simulink library "HDL_ieee_8021513"  (R2024a)
settings: Solver=FixedStepDiscrete  StartTime=0.0  StopTime=10.0  RelTol=1e-3
undefined symbols (not defined in the file or in its folder): Add, axiWidth, channelCyclicPrefixLen, channelDataCarriers, channelEstReference, channelLUT, channelOFDMSamples, channelScramblerInit, decimatorDelay, decimatorFilter, fPHY, frequencyOffsetTimeWindow, fs, headerBitsPerFec, headerBitsPerOFDMSymbol, headerBitsPerSubcarrier, headerCyclicPrefixLen, headerDataCarriers, headerOFDMSamples, headerScramblerInit, interpolatorDelay, interpolatorFilter, leftGuard, N, ncoCarrierFrequency, ncoWordLength, numDataCarriers, oversamplingFactor, payloadBitsPerFec, payloadScramblerInit, payloadWordsPerBlock0, peakDetectorThreshold, peakDetectorWindow, preambleCyclicPrefixLen, preambleDataCarriers, preambleLUT, preambleOFDMSamples, preambleScramblerInit, QAM, rightGuard, Shift
libraries: hdlsllib x198, $bdroot x80, whdlutilities x28, whdledac x10, whdlmod x7, simulink x4, dsphdlfiltering2 x2, dsphdlsigops2 x2, commhdlcrc x2, dspsigops x2, dspstat3 x2, commdigbbndam3 x2
(part 4 of 5)

== system HDL_ieee_8021513/full_rx/header_clock_x2 ==
  data_in : Inport
  valid_header : Inport  Port=2
  Demux : Demux
  Serializer1D : hdlsllib/HDL Operations/Serializer1D  Ratio=2  IdleCycles=0  validIn=on  startOut=off  validOut=on  inputDataDimensions=-1  inputSampleTime=-1  inputSignalType=auto
  Terminator : Terminator
  Terminator1 : Terminator
  Vector Concatenate : Concatenate  Mode=Multidimensional array  ConcatenateDimension=2
  rising_edge_detector : $bdroot/rising_edge_detector  SystemSampleTime=-1  VariantActivationTime=update diagram  AllowFlexibleInterface=on  Latency=0  AutoFrameSizeCalculation=off
  data_out : Outport
  start : Outport  Port=2
  wires:
  rising_edge_detector/1 -> start/1
  valid_header/1 -> Serializer1D/2
  data_in/1 -> Demux/1
  Demux/1 -> Terminator/1
  Demux/2 -> Terminator1/1
  Demux/3 -> Vector Concatenate/1
  Demux/4 -> Vector Concatenate/2
  Serializer1D/1 -> data_out/1
  Serializer1D/2 -> rising_edge_detector/1
  Vector Concatenate/1 -> Serializer1D/1

== system HDL_ieee_8021513/full_rx/prepare_payload_data ==
  note: Note_ this counter makes sure that the fifo always has data, and is not emptied in the middle of an LDPC block
  note: Maximum value is 3741
  data_in : Inport
  valid_payload : Inport  Port=2
  payload_ready : Inport  Port=3
  Delay : Delay  DelayLength=1  InitialCondition=0  UseCircularBuffer=on
  Delay2 : Delay  DelayLength=1  InitialCondition=0  UseCircularBuffer=on
  HDL Counter1 : hdlsllib/Sources/HDL Counter  CountType=Count limited  CountInit=0  CountStep=1  CountMax=10000  CountFromType=Initial value  CountFrom=0  CountResetPort=off  CountLoadPort=off  CountEnbPort=on  CountDirPort=off  CountHitOutputPort=on  CountDataType=Unsigned  CountWordLen=14  CountFracLen=0  CountSampTime=1
  HDL FIFO : hdlsllib/HDL RAMs/HDL FIFO  fifo_size=4096  mode=Classic  ratio=1/2  push_msg=Error  pop_msg=Error  show_empty=on  show_full=off  show_num=on  LabelModeActiveChoice_Mode=Classic  rst_port=off
  Logical Operator2 : Logic  IconShape=distinctive  AllPortsSameDT=off  OutDataTypeStr=boolean
  Logical Operator3 : Logic  Operator=NOT  IconShape=distinctive  AllPortsSameDT=off  OutDataTypeStr=boolean
  OR1 : Logic  Operator=OR  IconShape=distinctive  AllPortsSameDT=off  OutDataTypeStr=boolean
  Switch1 : Switch  Criteria=u2 ~= 0  SaturateOnIntegerOverflow=off  InputSameDT=off
  Terminator : Terminator
  Terminator1 : Terminator
  Unit Delay1 : UnitDelay  SampleTime=-1  HasFrameUpgradeWarning=on
  falling_edge_detector1 : $bdroot/falling_edge_detector  SystemSampleTime=-1  VariantActivationTime=update diagram  AllowFlexibleInterface=on  Latency=0  AutoFrameSizeCalculation=off
  payload_clock_x2 : Subsystem
  rising_edge_detector1 : $bdroot/rising_edge_detector  SystemSampleTime=-1  VariantActivationTime=update diagram  AllowFlexibleInterface=on  Latency=0  AutoFrameSizeCalculation=off
  dataOut : Outport
  valid_in : Outport  Port=2
  last_frame : Outport  Port=3
  new_frame : Outport  Port=4
  wires:
  HDL FIFO/3 -> Terminator/1  "fifo_count"
  Delay2/1 -> OR1/2
  HDL Counter1/1 -> Terminator1/1
  OR1/1 -> Switch1/2
  falling_edge_detector1/1 -> OR1/1, Switch1/1
  rising_edge_detector1/1 -> last_frame/1
  HDL Counter1/2 -> Delay2/1, new_frame/1  "new_frame"
  Unit Delay1/1 -> Switch1/3
  Switch1/1 -> HDL Counter1/1, Unit Delay1/1
  HDL FIFO/2 -> Logical Operator3/1, falling_edge_detector1/1, rising_edge_detector1/1  "fifo_empty"
  data_in/1 -> payload_clock_x2/1(data_in)
  payload_clock_x2/2(valid_out) -> HDL FIFO/2  "push"
  payload_clock_x2/1(data_out) -> HDL FIFO/1  "dataIn"
  HDL FIFO/1 -> dataOut/1  "dataOut"
  valid_payload/1 -> payload_clock_x2/2(valid_in)
  Logical Operator2/1 -> HDL FIFO/3, Delay/1
  Delay/1 -> valid_in/1  "valid_in"
  Logical Operator3/1 -> Logical Operator2/1
  payload_ready/1 -> Logical Operator2/2  "payload_ready"

== system HDL_ieee_8021513/full_tx/FIFO ==
  preamble : Inport
  preamble_valid : Inport  Port=2
  channel : Inport  Port=3
  channel_valid : Inport  Port=4
  header : Inport  Port=5
  header_valid : Inport  Port=6
  payload : Inport  Port=7
  payload_valid : Inport  Port=8
  payload_len : Inport  Port=9
  bits_per_subcarrier : Inport  Port=10
  cp_len_in : Inport  Port=11
  ready : Inport  Port=12
  Delay : Delay  DelayLength=1  InitialCondition=0  UseCircularBuffer=on
  HDL FIFO : hdlsllib/HDL RAMs/HDL FIFO  fifo_size=65536  mode=Classic  ratio=1  push_msg=Warning  pop_msg=Warning  show_empty=on  show_full=on  show_num=on  LabelModeActiveChoice_Mode=Classic  rst_port=off
  data_out : Outport
  valid_out : Outport  Port=2
  bits_per_subcarrier_out : Outport  Port=3
  init : Outport  Port=4
  new : Outport  Port=5
  cp_len : Outport  Port=6
  wires:
  Delay/1 -> valid_out/1
  HDL FIFO/1 -> data_out/1
  ready/1 -> HDL FIFO/3, Delay/1

== system HDL_ieee_8021513/full_tx/clock_crossing ==
  preamble_in : Inport
  preamble_ctrl_in : Inport  Port=2
  channel : Inport  Port=3
  channel_ctrl : Inport  Port=4
  header_in : Inport  Port=5
  header_ctrl_in : Inport  Port=6
  payload_in : Inport  Port=7
  payload_ctrl_in : Inport  Port=8
  cp_len_in : Inport  Port=9
  payload_len_in : Inport  Port=10
  bits_per_subcarrier_in : Inport  Port=11
  Deserializer1D : hdlsllib/HDL Operations/Deserializer1D  Ratio=2  IdleCycles=0  InitialCondition=0  startIn=off  validIn=on  validOut=on  inputDataDimensions=-1  inputSampleTime=-1  inputSignalType=auto
  Deserializer1D1 : hdlsllib/HDL Operations/Deserializer1D  Ratio=2  IdleCycles=0  InitialCondition=0  startIn=off  validIn=on  validOut=on  inputDataDimensions=-1  inputSampleTime=-1  inputSignalType=auto
  Rate Transition : RateTransition  OutPortSampleTime=1/fPHY
  Rate Transition1 : RateTransition  OutPortSampleTime=1/fPHY
  Rate Transition2 : RateTransition  OutPortSampleTime=1/fPHY
  Sample Control Bus Selector{,1..3} (4 alike) : whdlutilities/Sample Control Bus Selector  OutputSignals=start,end,valid
  Terminator{,1..7} (8 alike) : Terminator
  preamble_out : Outport
  preamble_valid : Outport  Port=2
  channel_out : Outport  Port=3
  channel_valid : Outport  Port=4
  header_out : Outport  Port=5
  header_valid : Outport  Port=6
  payload_out : Outport  Port=7
  payload_valid_out : Outport  Port=8
  payload_len_out : Outport  Port=9  VectorParamsAs1DForOutWhenUnconnected=off
  bits_per_subcarrier_out : Outport  Port=10  VectorParamsAs1DForOutWhenUnconnected=off
  cp_len_out : Outport  Port=11  VectorParamsAs1DForOutWhenUnconnected=off
  wires:
  preamble_ctrl_in/1 -> Sample Control Bus Selector/1
  Sample Control Bus Selector/1 -> Terminator/1
  Sample Control Bus Selector/2 -> Terminator1/1
  Sample Control Bus Selector/3 -> preamble_valid/1
  preamble_in/1 -> preamble_out/1
  Sample Control Bus Selector1/3 -> channel_valid/1
  channel_ctrl/1 -> Sample Control Bus Selector1/1
  Sample Control Bus Selector1/2 -> Terminator3/1
  Sample Control Bus Selector1/1 -> Terminator2/1
  channel/1 -> channel_out/1
  Sample Control Bus Selector2/1 -> Terminator5/1
  Deserializer1D/1 -> header_out/1
  Sample Control Bus Selector2/2 -> Terminator4/1
  Deserializer1D/2 -> header_valid/1
  header_ctrl_in/1 -> Sample Control Bus Selector2/1
  Sample Control Bus Selector2/3 -> Deserializer1D/2
  header_in/1 -> Deserializer1D/1
  Sample Control Bus Selector3/1 -> Terminator7/1
  Deserializer1D1/2 -> payload_valid_out/1
  Sample Control Bus Selector3/2 -> Terminator6/1
  payload_ctrl_in/1 -> Sample Control Bus Selector3/1
  Deserializer1D1/1 -> payload_out/1
  Sample Control Bus Selector3/3 -> Deserializer1D1/2
  payload_in/1 -> Deserializer1D1/1
  bits_per_subcarrier_in/1 -> Rate Transition2/1
  payload_len_in/1 -> Rate Transition1/1
  cp_len_in/1 -> Rate Transition/1
  Rate Transition/1 -> cp_len_out/1
  Rate Transition1/1 -> payload_len_out/1
  Rate Transition2/1 -> bits_per_subcarrier_out/1

== system HDL_ieee_8021513/full_tx/new_frame_rate_conversion ==
  note: Description:
      | This block "extends" the "end" signal 4 clock cycles, to ensure that the "end" signal can be sampled by the rate transition block.
      | (Otherwise, the "end" signal would be "on" only 1/4th of a cycle, and it can't be ensured that it will be read).
  ctrl_in : Inport
  Delay2 : Delay  DelayLength=1  InitialCondition=0  UseCircularBuffer=on
  Delay3 : Delay  DelayLength=1  InitialCondition=0  UseCircularBuffer=on
  Delay4 : Delay  DelayLength=1  InitialCondition=0  UseCircularBuffer=on
  Logical Operator : Logic  Operator=OR  Inputs=4  IconShape=distinctive  AllPortsSameDT=off  OutDataTypeStr=boolean
  Rate Transition2 : RateTransition  OutPortSampleTime=1/(fPHY/4)
  Sample Control Bus Selector1 : whdlutilities/Sample Control Bus Selector  OutputSignals=start,end,valid
  Terminator2 : Terminator
  Terminator3 : Terminator
  new_frame : Outport  VectorParamsAs1DForOutWhenUnconnected=off
  wires:
  Logical Operator/1 -> Rate Transition2/1
  Sample Control Bus Selector1/3 -> Terminator2/1
  Delay2/1 -> Logical Operator/2, Delay3/1
  Delay3/1 -> Logical Operator/3, Delay4/1
  Sample Control Bus Selector1/2 -> Logical Operator/1, Delay2/1
  Delay4/1 -> Logical Operator/4
  Sample Control Bus Selector1/1 -> Terminator3/1
  ctrl_in/1 -> Sample Control Bus Selector1/1
  Rate Transition2/1 -> new_frame/1

== system HDL_ieee_8021513/full_tx/new_frame_rate_conversion1 ==
  note: Description:
      | This block "extends" the "end" signal 8 clock cycles, to ensure that the "end" signal can be sampled by the rate transition block.
      | (Otherwise, the "end" signal would be "on" only 1/4th of a cycle, and it can't be ensured that it will be read).
  ctrl_in : Inport
  Delay{1..7} (7 alike) : Delay  DelayLength=1  InitialCondition=0  UseCircularBuffer=on
  Logical Operator : Logic  Operator=OR  Inputs=8  IconShape=distinctive  AllPortsSameDT=off  OutDataTypeStr=boolean
  Rate Transition2 : RateTransition  OutPortSampleTime=1/(fPHY/4)
  Sample Control Bus Selector1 : whdlutilities/Sample Control Bus Selector  OutputSignals=start,end,valid
  Terminator2 : Terminator
  Terminator3 : Terminator
  new_frame : Outport  VectorParamsAs1DForOutWhenUnconnected=off
  wires:
  Logical Operator/1 -> Rate Transition2/1
  Sample Control Bus Selector1/3 -> Terminator2/1
  Delay2/1 -> Logical Operator/2, Delay3/1
  Delay3/1 -> Logical Operator/3, Delay4/1
  Sample Control Bus Selector1/2 -> Logical Operator/1, Delay2/1
  Delay4/1 -> Logical Operator/8, Delay1/1
  Sample Control Bus Selector1/1 -> Terminator3/1
  ctrl_in/1 -> Sample Control Bus Selector1/1
  Rate Transition2/1 -> new_frame/1
  Delay1/1 -> Logical Operator/7, Delay5/1
  Delay5/1 -> Logical Operator/6, Delay6/1
  Delay6/1 -> Logical Operator/5, Delay7/1
  Delay7/1 -> Logical Operator/4

== system HDL_ieee_8021513/full_tx/store_frame_in_ram ==
  preamble : Inport
  preamble_valid : Inport  Port=2
  channel : Inport  Port=3
  channel_valid : Inport  Port=4
  header : Inport  Port=5
  header_valid : Inport  Port=6
  payload : Inport  Port=7
  payload_valid : Inport  Port=8
  payload_len : Inport  Port=9
  bits_per_subcarrier : Inport  Port=10
  cp_len_in : Inport  Port=11
  ready : Inport  Port=12
  Delay : Delay  DelayLength=1  InitialCondition=0  UseCircularBuffer=on
  RAM : Subsystem
  Switch1 : Switch  Criteria=u2 ~= 0  SaturateOnIntegerOverflow=off  InputSameDT=off
  Unit Delay1 : UnitDelay  SampleTime=-1  HasFrameUpgradeWarning=on
  read_frame_from_ram : Subsystem
  write_frame_to_ram : Subsystem
  data_out : Outport
  valid_out : Outport  Port=2
  bits_per_subcarrier_out : Outport  Port=3
  init : Outport  Port=4
  new : Outport  Port=5
  cp_len : Outport  Port=6
  wires:
  read_frame_from_ram/1(rd_addr) -> RAM/4(new_rd_addr)  "new_rd_addr"
  bits_per_subcarrier/1 -> read_frame_from_ram/3(bits_per_subcarrier)
  header/1 -> write_frame_to_ram/5(header)
  write_frame_to_ram/1(write_data) -> RAM/1(new_din)  "new_din"
  write_frame_to_ram/4(end) -> read_frame_from_ram/1(start_reading)
  cp_len_in/1 -> read_frame_from_ram/4(cp_len_in)
  Switch1/1 -> Unit Delay1/1, data_out/1  "dout_magic"
  write_frame_to_ram/3(we) -> RAM/3(new_we)  "new_we"
  ready/1 -> read_frame_from_ram/Enable, Delay/1
  Delay/1 -> Switch1/2
  preamble/1 -> write_frame_to_ram/1(preamble)
  channel_valid/1 -> write_frame_to_ram/4(channel_valid)
  read_frame_from_ram/3(bits_per_subcarrier_out) -> bits_per_subcarrier_out/1
  payload/1 -> write_frame_to_ram/7(payload)
  RAM/1(dout_new) -> Switch1/1
  read_frame_from_ram/5(new) -> new/1  "new_new"
  read_frame_from_ram/4(init) -> init/1
  write_frame_to_ram/5(ram_size) -> read_frame_from_ram/2(ram_size)
  preamble_valid/1 -> write_frame_to_ram/2(preamble_valid)
  Unit Delay1/1 -> Switch1/3
  payload_len/1 -> write_frame_to_ram/9(payload_len)
  channel/1 -> write_frame_to_ram/3(channel)
  write_frame_to_ram/2(wr_addr) -> RAM/2(new_wr_addr)  "new_wr_addr"
  read_frame_from_ram/2(valid_out) -> valid_out/1  "valid_new"
  payload_valid/1 -> write_frame_to_ram/8(payload_valid)
  header_valid/1 -> write_frame_to_ram/6(header_valid)
  read_frame_from_ram/6(cp_len) -> cp_len/1

== system HDL_ieee_8021513/ldpc_encoder/output_selector ==
  codeRate : Inport
  blockSize : Inport  Port=2
  Buffer1 : $bdroot/Buffer  SystemSampleTime=-1  VariantActivationTime=update diagram  AllowFlexibleInterface=on  Latency=0  AutoFrameSizeCalculation=off
  Demux2 : Demux  Outputs=2
  Demux3 : Demux  Outputs=3
  Logical Operator3 : Logic  IconShape=distinctive  AllPortsSameDT=off  OutDataTypeStr=boolean
  Logical Operator5 : Logic  Operator=OR  IconShape=distinctive  AllPortsSameDT=off  OutDataTypeStr=boolean
  Logical Operator6 : Logic  IconShape=distinctive  AllPortsSameDT=off  OutDataTypeStr=boolean
  Logical Operator7 : Logic  Operator=NOT  IconShape=distinctive  AllPortsSameDT=off  OutDataTypeStr=boolean
  Terminator1 : Terminator
  m2 : Outport  VectorParamsAs1DForOutWhenUnconnected=off
  m1 : Outport  Port=2  VectorParamsAs1DForOutWhenUnconnected=off
  m0 : Outport  Port=3  VectorParamsAs1DForOutWhenUnconnected=off
  wires:
  Buffer1/1 -> m0/1  "Out0"
  Logical Operator6/1 -> m1/1  "Out1"
  codeRate/1 -> Demux3/1
  blockSize/1 -> Demux2/1
  Demux2/1 -> Buffer1/1  "K0"
  Demux3/1 -> Logical Operator3/2, Logical Operator7/1  "R0"
  Logical Operator5/1 -> m2/1  "Out2"
  Logical Operator7/1 -> Logical Operator6/1
  Demux3/2 -> Logical Operator6/2, Logical Operator3/1  "R1"
  Demux2/2 -> Terminator1/1  "K1"
  Logical Operator3/1 -> Logical Operator5/1
  Demux3/3 -> Logical Operator5/2  "R2"

== system HDL_ieee_8021513/ofdm_separator/wait_for_header ==
  note: Store payload OFDM symbols until header parameters are known (cyclic prefix has to be known before demodulating the OFDM symbol)
  note: The RAM value should be large enough to wait for the header to be processed.
      | Th e LDPC decoder of the header has a delay > 2500, so a value of 3000 is chosen for an extra margin.
  data_in : Inport
  header_ready : Inport  Port=2
  valid_payload : Inport  Port=3
  zero_payload : Inport  Port=4
  one_payload : Inport  Port=5
  ofdm_samples : Inport  Port=6
  AND : Logic  IconShape=distinctive  AllPortsSameDT=off  OutDataTypeStr=boolean
  Delay12 : Delay  DelayLength=1  InitialCondition=0  UseCircularBuffer=on
  Delay13 : Delay  DelayLength=1  InitialCondition=0  UseCircularBuffer=on
  Delay14 : Delay  DelayLength=1  InitialCondition=0  UseCircularBuffer=on
  HDL Counter : hdlsllib/Sources/HDL Counter  CountType=Free running  CountInit=0  CountStep=1  CountMax=25  CountFromType=Initial value  CountFrom=0  CountResetPort=on  CountLoadPort=off  CountEnbPort=on  CountDirPort=off  CountHitOutputPort=off  CountDataType=Unsigned  CountWordLen=16  CountFracLen=0  CountSampTime=1
  HDL FIFO : hdlsllib/HDL RAMs/HDL FIFO  fifo_size=2100  mode=Classic  ratio=1  push_msg=Error  pop_msg=Error  show_empty=on  show_full=off  show_num=on  LabelModeActiveChoice_Mode=Classic  rst_port=on
  Logical Operator1 : Logic  Operator=OR  Inputs=3  IconShape=distinctive  AllPortsSameDT=off  OutDataTypeStr=boolean
  NOT : Logic  Operator=NOT  IconShape=distinctive  AllPortsSameDT=off  OutDataTypeStr=boolean
  OR : Logic  Operator=OR  IconShape=distinctive  AllPortsSameDT=off  OutDataTypeStr=boolean
  OR2 : Logic  Operator=OR  IconShape=distinctive  AllPortsSameDT=off  OutDataTypeStr=boolean
  Relational Operator : RelationalOperator  Operator===  OutDataTypeStr=boolean  RndMeth=Simplest  InputSameDT=off
  Switch : Switch  Criteria=u2 ~= 0  SaturateOnIntegerOverflow=off  InputSameDT=off
  Switch3 : Switch  Criteria=u2 ~= 0  SaturateOnIntegerOverflow=off  InputSameDT=off
  Terminator : Terminator
  Unit Delay : UnitDelay  SampleTime=-1  HasFrameUpgradeWarning=on
  rising_edge_detector : $bdroot/rising_edge_detector  SystemSampleTime=-1  VariantActivationTime=update diagram  AllowFlexibleInterface=on  Latency=0  AutoFrameSizeCalculation=off
  rising_edge_detector1 : $bdroot/rising_edge_detector  SystemSampleTime=-1  VariantActivationTime=update diagram  AllowFlexibleInterface=on  Latency=0  AutoFrameSizeCalculation=off
  data_out : Outport
  valid_payload_out : Outport  Port=2
  wires:
  Delay13/1 -> HDL FIFO/2
  data_in/1 -> Switch3/3, Delay12/1
  Delay12/1 -> HDL FIFO/1
  valid_payload/1 -> Delay13/1, rising_edge_detector1/1
  Switch3/1 -> data_out/1
  HDL FIFO/2 -> [empty]
  HDL FIFO/1 -> Switch3/1
  rising_edge_detector1/1 -> OR/1
  zero_payload/1 -> OR/2
  HDL FIFO/3 -> Terminator/1  "fifo_ofdm"
  [empty] -> rising_edge_detector/1
  rising_edge_detector/1 -> Logical Operator1/1
  Unit Delay/1 -> Switch/3
  Switch/1 -> Delay14/1, HDL FIFO/3, Unit Delay/1  "pop"
  Logical Operator1/1 -> Switch/2
  header_ready/1 -> HDL Counter/1, Switch/1, Logical Operator1/2
  HDL Counter/1 -> Relational Operator/1  "count"
  ofdm_samples/1 -> Relational Operator/2
  OR/1 -> OR2/1
  Relational Operator/1 -> OR2/2, NOT/1, Logical Operator1/3  "hit_zero"
  OR2/1 -> HDL FIFO/4
  one_payload/1 -> HDL Counter/2
  AND/1 -> Switch3/2, valid_payload_out/1
  Delay14/1 -> AND/1
  NOT/1 -> AND/2

== system HDL_ieee_8021513/ofdm_symbol_sync/find_peak ==
  data_in : Inport
  M_in : Inport  Port=2
  Compare To Constant : hdlsllib/Logic and Bit Operations/Compare To Constant  relop=>  const=peakDetectorThreshold  OutDataTypeStr=boolean
  Constant : Constant  Value=0  OutDataTypeStr=Inherit: Inherit via back propagation  SampleTime=-1
  Delay{,1..4} (5 alike) : Delay  DelayLength=1  InitialCondition=0  UseCircularBuffer=on
  Delay5 : Delay  DelayLength=peakDetectorWindow-1  InitialCondition=0  UseCircularBuffer=on
  HDL Counter : hdlsllib/Sources/HDL Counter  CountType=Count limited  CountInit=0  CountStep=1  CountMax=peakDetectorWindow-1  CountFromType=Initial value  CountFrom=0  CountResetPort=on  CountLoadPort=off  CountEnbPort=on  CountDirPort=off  CountHitOutputPort=on  CountDataType=Unsigned  CountWordLen=nextpow2(peakDetectorWindow)  CountFracLen=0  CountSampTime=1
  OR : Logic  Operator=OR  IconShape=distinctive  AllPortsSameDT=off  OutDataTypeStr=boolean
  OR1 : Logic  Operator=OR  IconShape=distinctive  AllPortsSameDT=off  OutDataTypeStr=boolean
  Relational Operator : RelationalOperator  Operator=>  OutDataTypeStr=boolean  InputSameDT=off
  Switch : Switch  Criteria=u2 ~= 0  SaturateOnIntegerOverflow=off
  Switch1 : Switch  Criteria=u2 ~= 0  SaturateOnIntegerOverflow=off
  Switch2 : Switch  Criteria=u2 ~= 0  SaturateOnIntegerOverflow=off  InputSameDT=off
  Terminator : Terminator
  Unit Delay : UnitDelay  SampleTime=-1  HasFrameUpgradeWarning=on
  Unit Delay1 : UnitDelay  SampleTime=-1  HasFrameUpgradeWarning=on
  data_out : Outport  VectorParamsAs1DForOutWhenUnconnected=off
  peak_sync : Outport  Port=2  VectorParamsAs1DForOutWhenUnconnected=off
  wires:
  M_in/1 -> Switch1/1, Compare To Constant/1  "data_in"
  Unit Delay/1 -> Switch/3
  Switch/1 -> Unit Delay/1, Relational Operator/2  "peak(i)"
  Relational Operator/1 -> HDL Counter/1, Delay3/1  "new_peak"
  Switch1/1 -> Delay2/1  "peak(i+1)"
  Constant/1 -> Switch1/3
  Unit Delay1/1 -> Switch2/3
  Switch2/1 -> Unit Delay1/1, HDL Counter/2  "en"
  HDL Counter/2 -> Delay1/1, peak_sync/1
  OR/1 -> Switch2/2
  [new_peak] -> OR/2
  [peak_found] -> OR/1
  HDL Counter/1 -> Terminator/1
  Delay/1 -> Switch/1
  Delay1/1 -> [peak_found]  "peak_found"
  OR1/1 -> Switch/2
  [new_peak] -> OR1/1
  [peak_found] -> OR1/2
  Delay3/1 -> [new_peak], Switch2/1
  Compare To Constant/1 -> Switch1/2
  Delay2/1 -> Delay/1, Relational Operator/1
  data_in/1 -> Delay4/1
  Delay4/1 -> Delay5/1
  Delay5/1 -> data_out/1

== system HDL_ieee_8021513/ofdm_symbol_sync/frequency_offset_calculator ==
  peak_sync : Inport
  P(d) : Inport  Port=2
  Complex to Magnitude-Angle : dsphdlmathfun2/Complex to Magnitude-Angle  NumIterationsSource=Auto  NumIterations=10  OutputFormat=Angle  AngleFormat=Radians  ScaleOutput=off  ScalingMethod=Shift-Add  SimulateUsing=Code generation
  Delay : Delay  InitialCondition=0  UseCircularBuffer=on
  Delay1 : Delay  InitialCondition=0  UseCircularBuffer=on
  Gain : Gain  Gain=fi(1/(pi*frequencyOffsetTimeWindow), 0, 32, 16)  ParamDataTypeStr=fixdt(0,32,16)  OutDataTypeStr=fixdt(1,32,16)
  Switch : Switch  Criteria=u2 ~= 0  SaturateOnIntegerOverflow=off  InputSameDT=off
  Unit Delay : UnitDelay  SampleTime=-1  HasFrameUpgradeWarning=on
  frequency_offset : Outport
  wires:
  Switch/1 -> Unit Delay/1, frequency_offset/1
  Unit Delay/1 -> Switch/3
  Delay/1 -> Switch/1
  Delay1/1 -> Switch/2
  Gain/1 -> Delay/1
  Complex to Magnitude-Angle/1 -> Gain/1
  P(d)/1 -> Complex to Magnitude-Angle/1
  peak_sync/1 -> Complex to Magnitude-Angle/2
  Complex to Magnitude-Angle/2 -> Delay1/1

== system HDL_ieee_8021513/ofdm_symbol_sync/m_cox ==
  note: Latency of the real divide block is:
      |
      | 1 + nextpow2(u.WordLength + 1 - issigned(u) + 1) + 2 + u.WordLength + 2 - issigned(u) + 5
  note: Delay of m_cox = delay blocks + delay divider + delay_10_preambles_symbols
      | Delay of m_cox = 5 + 47 + 2580
  data_in : Inport
  Compare To Zero : hdlsllib/Logic and Bit Operations/Compare To Zero  relop=~=  OutDataTypeStr=boolean
  Constant : Constant  OutDataTypeStr=boolean  SampleTime=-1
  Constant1 : Constant  OutDataTypeStr=Inherit: Inherit via back propagation  SampleTime=-1
  Data Type Conversion1 : DataTypeConversion  OutDataTypeStr=fixdt(1,32,24)  SaturateOnIntegerOverflow=off  RndMeth=Floor
  Delay1 : Delay  DelayLength=47  InitialCondition=0  UseCircularBuffer=on
  Delay4 : Delay  DelayLength=(N+preambleCyclicPrefixLen)*10  InitialCondition=0  UseCircularBuffer=on
  Delay5 : Delay  DelayLength=47  InitialCondition=0  UseCircularBuffer=on
  Delay6 : Delay  DelayLength=5  InitialCondition=0  UseCircularBuffer=on
  Real Divide HDL Optimized : embreciprocals/Real Divide HDL Optimized  OutputType=fixdt(1,16,12)
      settings: LibrarySourceBlock=embeddedMatrixLib/Math Operations/Real Divide HDL Optimized
  Switch : Switch  Criteria=u2 ~= 0  SaturateOnIntegerOverflow=off  InputSameDT=off
  Terminator : Terminator
  calculate_P : Subsystem
  calculate_R : Subsystem
  data_out : Outport  VectorParamsAs1DForOutWhenUnconnected=off
  M(d) : Outport  Port=2  VectorParamsAs1DForOutWhenUnconnected=off
  P(d) : Outport  Port=3  VectorParamsAs1DForOutWhenUnconnected=off
  wires:
  Constant/1 -> Real Divide HDL Optimized/3
  data_in/1 -> Delay4/1, Data Type Conversion1/1
  calculate_P/1(|P(d)|2) -> Real Divide HDL Optimized/1  "P"
  Real Divide HDL Optimized/1 -> M(d)/1
  Delay1/1 -> P(d)/1
  Delay6/1 -> Delay5/1
  Delay5/1 -> data_out/1
  Delay4/1 -> Delay6/1
  calculate_P/2(P(d)) -> Delay1/1
  Data Type Conversion1/1 -> calculate_R/1(r(d)), calculate_P/1(r(d))
  Real Divide HDL Optimized/2 -> Terminator/1
  Constant1/1 -> Switch/3
  Compare To Zero/1 -> Switch/2
  Switch/1 -> Real Divide HDL Optimized/2
  calculate_R/1(Rf2) -> Switch/1, Compare To Zero/1  "R"

== system HDL_ieee_8021513/payload_full/psdu_size_to_payload_len ==
  note: Get length of the payload expressed in OFDM Symbols:
      |
      | bitsInPsdu = psduSize * 8 * fecRate [bits/payload]
      | bitsInOFDMSymbol = numDataCarriers * bitsPerSubcarrier [bits/OFDM]
      |
      | payloadLenInOFDMSymbols = ceil( bitsInPsdu / bitsInOFDMSymbol ) [OFDM/payload]
  note: Repetition not supported
  note: Adding "1" is the same as doing a "ceil()" operation,
      | because the divider "floors" the previous result.
      | It is assumed that the division will never be an integer
  bits_per_subcarrier : Inport
  psdu_size : Inport  Port=2
  rep_number : Inport  Port=3
  Add1 : Sum  OutDataTypeStr=Inherit: Same as first input
  Bit Shift : hdlsllib/Logic and Bit Operations/Bit Shift  mode=Shift Left Logical  N=4
  Bit Shift2 : hdlsllib/Logic and Bit Operations/Bit Shift  mode=Shift Right Arithmetic  N=0
  Bit Shift3 : hdlsllib/Logic and Bit Operations/Bit Shift  mode=Shift Right Arithmetic  N=1
  Bit Shift5 : hdlsllib/Logic and Bit Operations/Bit Shift  mode=Shift Right Arithmetic  N=4
  Bits to Word1 : hdlsllib/Logic and Bit Operations/Bits to Word
  Constant4 : Constant  OutDataTypeStr=fixdt(0,1,0)  SampleTime=-1
  Data Type Conversion1 : DataTypeConversion  OutDataTypeStr=fixdt(0,1,0)  SaturateOnIntegerOverflow=off  RndMeth=Floor
  Delay{,1..2,6} (4 alike) : Delay  DelayLength=1  InitialCondition=0  UseCircularBuffer=on
  Gain : Gain  Gain=fi(1/numDataCarriers, 0, 16, 16)  ParamDataTypeStr=fixdt(1,16,15)  OutDataTypeStr=uint16
  Multiport Switch : MultiPortSwitch  DataPortOrder=Zero-based contiguous  Inputs=5  zeroidx=on  SaturateOnIntegerOverflow=off  InputSameDT=off
  Terminator : Terminator
  payload_len_in_ofdm_symbols : Outport
  wires:
  rep_number/1 -> Terminator/1
  bits_per_subcarrier/1 -> Delay1/1
  Data Type Conversion1/1 -> Bits to Word1/1
  Multiport Switch/1 -> Gain/1
  Constant4/1 -> Add1/2
  psdu_size/1 -> Data Type Conversion1/1
  Bits to Word1/1 -> Bit Shift/1
  Add1/1 -> Delay6/1  "payloadNumOFDMSymbols"
  Delay6/1 -> payload_len_in_ofdm_symbols/1
  Bit Shift/1 -> Delay/1
  Bit Shift2/1 -> Multiport Switch/2, Multiport Switch/3
  Bit Shift3/1 -> Multiport Switch/5, Multiport Switch/4
  Bit Shift5/1 -> Multiport Switch/6
  Delay/1 -> Bit Shift2/1, Bit Shift5/1, Bit Shift3/1
  Delay1/1 -> Multiport Switch/1
  Gain/1 -> Delay2/1
  Delay2/1 -> Add1/1

== system HDL_ieee_8021513/peak_detector/local_peak ==
  index : Inport
  dataIn : Inport  Port=2
  AND : Logic  IconShape=distinctive  AllPortsSameDT=off  OutDataTypeStr=boolean
  AND1 : Logic  IconShape=distinctive  AllPortsSameDT=off  OutDataTypeStr=boolean
  AND2 : Logic  IconShape=distinctive  AllPortsSameDT=off  OutDataTypeStr=boolean
  Delay{,1..5} (6 alike) : Delay  DelayLength=1  InitialCondition=0  UseCircularBuffer=on
  HDL Counter : hdlsllib/Sources/HDL Counter  CountType=Count limited  CountInit=0  CountStep=1  CountMax=peakDetectorWindow-1  CountFromType=Initial value  CountFrom=0  CountResetPort=on  CountLoadPort=off  CountEnbPort=on  CountDirPort=off  CountHitOutputPort=on  CountDataType=Unsigned  CountWordLen=nextpow2(peakDetectorWindow+1)  CountFracLen=0  CountSampTime=-1
  NOT : Logic  Operator=NOT  IconShape=distinctive  AllPortsSameDT=off  OutDataTypeStr=boolean
  OR : Logic  Operator=OR  IconShape=distinctive  AllPortsSameDT=off  OutDataTypeStr=boolean
  OR1 : Logic  Operator=OR  IconShape=distinctive  AllPortsSameDT=off  OutDataTypeStr=boolean
  OR2 : Logic  Operator=OR  IconShape=distinctive  AllPortsSameDT=off  OutDataTypeStr=boolean
  Relational Operator : RelationalOperator  OutDataTypeStr=boolean  RndMeth=Simplest  InputSameDT=off
  Switch : Switch  Criteria=u2 ~= 0  SaturateOnIntegerOverflow=off  InputSameDT=off
  Switch1 : Switch  Criteria=u2 ~= 0  SaturateOnIntegerOverflow=off  InputSameDT=off
  Terminator : Terminator
  Unit Delay : UnitDelay  SampleTime=-1  HasFrameUpgradeWarning=on
  Unit Delay1 : UnitDelay  SampleTime=-1  HasFrameUpgradeWarning=on
  peak_sync : Outport
  wires:
  HDL Counter/1 -> Terminator/1  "count"
  Unit Delay/1 -> Switch/3
  Switch/1 -> Relational Operator/2, Unit Delay/1  "dataIn(indexes(i)"
  Unit Delay1/1 -> Switch1/3
  Switch1/1 -> HDL Counter/2, Delay3/1, Unit Delay1/1  "count_enable"
  OR/1 -> Delay4/1
  dataIn/1 -> Relational Operator/1, Delay1/1
  index/1 -> AND1/1  "input"
  Delay4/1 -> Switch1/2  "open"
  Delay5/1 -> Switch1/1  "new_index"
  Delay/1 -> Switch/2
  Delay1/1 -> Switch/1
  Relational Operator/1 -> [higher]
  NOT/1 -> AND1/2
  AND1/1 -> [new_peak], OR1/1
  OR1/1 -> Delay2/1  "rst"
  AND2/1 -> OR1/2
  AND/1 -> OR2/1
  OR2/1 -> Delay/1
  [en] -> NOT/1
  [en] -> AND2/1
  [en] -> AND/1
  Delay3/1 -> [en]
  [higher] -> AND/2
  [higher] -> AND2/2
  [peak_found] -> OR/2
  HDL Counter/2 -> peak_sync/1, [peak_found]  "counter_hit"
  [new_peak] -> Delay5/1
  [new_peak] -> OR/1
  [new_peak] -> OR2/2
  Delay2/1 -> HDL Counter/1  "new_index"

== system HDL_ieee_8021513/peak_detector/s1_index ==
  dataIn : Inport
  Add : Sum
  Bit Shift : hdlsllib/Logic and Bit Operations/Bit Shift  mode=Shift Right Arithmetic  N=1
  Compare To Constant : hdlsllib/Logic and Bit Operations/Compare To Constant  relop=>  const=peakDetectorThreshold  OutDataTypeStr=boolean
  Delay : Delay  DelayLength=peakDetectorWindow  InitialCondition=0  UseCircularBuffer=on
  Delay{1..5} (5 alike) : Delay  DelayLength=1  InitialCondition=0  UseCircularBuffer=on
  Minimum : dspstat3/Minimum  operation=minimum  fcn=Value  indexBase=Zero  operateOver=Each column  Dimension=1  InputProcessing=Columns as channels (frame based)  reset=None  roiEnable=off  roiType=Rectangles  roiPortion=Entire ROI  roiOutput=Individual statistics for each ROI  roiFlag=off  roundingMode=Floor  overflowMode=off
      settings: LibrarySourceBlock=dsphdlsupportstat/Minimum
  Minimum1 : dspstat3/Minimum  operation=minimum  fcn=Value  indexBase=Zero  operateOver=Each column  Dimension=1  InputProcessing=Columns as channels (frame based)  reset=None  roiEnable=off  roiType=Rectangles  roiPortion=Entire ROI  roiOutput=Individual statistics for each ROI  roiFlag=off  roundingMode=Floor  overflowMode=off
      settings: LibrarySourceBlock=dsphdlsupportstat/Minimum
  Tapped Delay : simulink/Discrete/Tapped Delay  vinit=0.0  samptime=-1  NumDelays=peakDetectorWindow  DelayOrder=Oldest  includeCurrent=off
  Tapped Delay1 : simulink/Discrete/Tapped Delay  vinit=0.0  samptime=-1  NumDelays=peakDetectorWindow  DelayOrder=Oldest  includeCurrent=off
  indexes : Outport
  Output : Outport  Port=2
  wires:
  dataIn/1 -> Tapped Delay/1, Delay/1  "x(i+peakDetectorWindow+1)"
  Delay/1 -> Delay2/1  "x(i+1)"
  Tapped Delay/1 -> Minimum/1  "x(i+1:i+peakDetectorWindow)"
  Tapped Delay1/1 -> Minimum1/1  "x(i-peakDetectorWindow:i-1)"
  Minimum/1 -> Add/1  "xmin_new"
  Minimum1/1 -> Add/2  "xmin_bot"
  Bit Shift/1 -> Delay3/1  "s1"
  Delay2/1 -> Delay4/1, Tapped Delay1/1  "x(i)"
  Compare To Constant/1 -> indexes/1
  Add/1 -> Delay1/1
  Delay1/1 -> Bit Shift/1
  Delay3/1 -> Compare To Constant/1
  Delay4/1 -> Delay5/1
  Delay5/1 -> Output/1

== system HDL_ieee_8021513/qam_demod/to_12bit_integer ==
  1bit : Inport
  2bit : Inport  Port=2
  4bit : Inport  Port=3
  Constant{,1..2,12,14} (5 alike) : Constant  Value=0  OutDataTypeStr=Inherit: Inherit via back propagation  SampleTime=-1
  Demux : Demux  Outputs=2
  Demux1 : Demux
  Vector Concatenate : Concatenate  NumInputs=4  Mode=Multidimensional array
  Vector Concatenate1 : Concatenate  NumInputs=4  Mode=Multidimensional array
  Vector Concatenate2 : Concatenate  NumInputs=4  Mode=Multidimensional array
  1bit_out : Outport
  2bit_out : Outport  Port=2
  4bit_out : Outport  Port=3
  wires:
  2bit/1 -> Demux/1
  4bit/1 -> Demux1/1
  Vector Concatenate/1 -> 4bit_out/1
  Vector Concatenate1/1 -> 2bit_out/1
  Vector Concatenate2/1 -> 1bit_out/1
  Constant2/1 -> Vector Concatenate2/1
  Constant1/1 -> Vector Concatenate2/2
  Constant/1 -> Vector Concatenate2/3
  1bit/1 -> Vector Concatenate2/4
  Constant14/1 -> Vector Concatenate1/1
  Constant12/1 -> Vector Concatenate1/2
  Demux/1 -> Vector Concatenate1/3
  Demux/2 -> Vector Concatenate1/4
  Demux1/1 -> Vector Concatenate/1
  Demux1/2 -> Vector Concatenate/2
  Demux1/3 -> Vector Concatenate/3
  Demux1/4 -> Vector Concatenate/4

== system HDL_ieee_8021513/rx_demodulator_full/get_bits_per_subcarrier ==
  payload_bits_per_sub : Inport
  valid_header : Inport  Port=2
  Constant3 : Constant  Value=headerBitsPerSubcarrier  OutDataTypeStr=uint8  SampleTime=-1
  Data Type Conversion2 : DataTypeConversion  OutDataTypeStr=fixdt(0,4,0)  SaturateOnIntegerOverflow=off  RndMeth=Floor
  Data Type Conversion7 : DataTypeConversion  OutDataTypeStr=fixdt(0,4,0)  SaturateOnIntegerOverflow=off  RndMeth=Floor
  Switch1 : Switch  Criteria=u2 ~= 0  SaturateOnIntegerOverflow=off  InputSameDT=off
  qam_demod_bits : Outport
  wires:
  Switch1/1 -> qam_demod_bits/1
  payload_bits_per_sub/1 -> Data Type Conversion2/1
  valid_header/1 -> Switch1/2
  Data Type Conversion2/1 -> Switch1/3
  Constant3/1 -> Data Type Conversion7/1
  Data Type Conversion7/1 -> Switch1/1

== system HDL_ieee_8021513/rx_demodulator_full/get_cp ==
  valid_header : Inport
  valid_payload : Inport  Port=2
  cp_payload : Inport  Port=3
  Bit Concat : hdlsllib/Logic and Bit Operations/Bit Concat  numInputs=2
  Constant : Constant  Value=channelCyclicPrefixLen  OutDataTypeStr=uint8  SampleTime=-1
  Constant1 : Constant  Value=headerCyclicPrefixLen  OutDataTypeStr=uint8  SampleTime=-1
  Data Type Conversion : DataTypeConversion  OutDataTypeStr=uint8  SaturateOnIntegerOverflow=off  RndMeth=Floor
  Data Type Conversion1 : DataTypeConversion  OutDataTypeStr=fixdt(0,2,0)  SaturateOnIntegerOverflow=off  RndMeth=Floor
  Data Type Conversion5 : DataTypeConversion  OutDataTypeStr=uint8  SaturateOnIntegerOverflow=off  RndMeth=Floor
  Data Type Conversion6 : DataTypeConversion  OutDataTypeStr=uint8  SaturateOnIntegerOverflow=off  RndMeth=Floor
  Multiport Switch : MultiPortSwitch  DataPortOrder=Zero-based contiguous  zeroidx=on  SaturateOnIntegerOverflow=off
  ofdm_cp_len : Outport
  wires:
  Data Type Conversion1/1 -> Multiport Switch/1
  valid_header/1 -> Bit Concat/2
  valid_payload/1 -> Bit Concat/1
  Data Type Conversion/1 -> Multiport Switch/4
  Data Type Conversion5/1 -> Multiport Switch/3
  Data Type Conversion6/1 -> Multiport Switch/2
  Multiport Switch/1 -> ofdm_cp_len/1
  cp_payload/1 -> Data Type Conversion/1
  Constant/1 -> Data Type Conversion6/1
  Constant1/1 -> Data Type Conversion5/1
  Bit Concat/1 -> Data Type Conversion1/1  "control"

== system HDL_ieee_8021513/rx_demodulator_full/get_init ==
  valid_header : Inport
  valid_payload : Inport  Port=2
  Bit Concat : hdlsllib/Logic and Bit Operations/Bit Concat  numInputs=2
  Constant4 : Constant  Value=channelScramblerInit  OutDataTypeStr=uint8  SampleTime=-1
  Constant5 : Constant  Value=headerScramblerInit  OutDataTypeStr=uint8  SampleTime=-1
  Constant6 : Constant  Value=payloadScramblerInit  OutDataTypeStr=uint8  SampleTime=-1
  Data Type Conversion10 : DataTypeConversion  OutDataTypeStr=boolean  SaturateOnIntegerOverflow=off  RndMeth=Floor
  Data Type Conversion4 : DataTypeConversion  OutDataTypeStr=boolean  SaturateOnIntegerOverflow=off  RndMeth=Floor
  Data Type Conversion9 : DataTypeConversion  OutDataTypeStr=boolean  SaturateOnIntegerOverflow=off  RndMeth=Floor
  Multiport Switch2 : MultiPortSwitch  DataPortOrder=Zero-based contiguous  zeroidx=on  SaturateOnIntegerOverflow=off  InputSameDT=off
  descrambler_init : Outport
  wires:
  Bit Concat/1 -> Multiport Switch2/1  "control"
  valid_header/1 -> Bit Concat/2
  valid_payload/1 -> Bit Concat/1
  Data Type Conversion10/1 -> Multiport Switch2/2
  Multiport Switch2/1 -> descrambler_init/1
  Constant4/1 -> Data Type Conversion10/1
  Constant5/1 -> Data Type Conversion9/1
  Data Type Conversion4/1 -> Multiport Switch2/4
  Constant6/1 -> Data Type Conversion4/1
  Data Type Conversion9/1 -> Multiport Switch2/3

== system HDL_ieee_8021513/rx_demodulator_full/ofdm_rx_counter ==
  note: Counts the amount of OFDM symbols for every "end" signal, and assigns them a position (preamble, channel, header, payload)
  valid : Inport
  rst : Inport  Port=2
  payload_num_ofdm_symbols : Inport  Port=3
  Add : Sum
  Constant1 : Constant  Value=2  OutDataTypeStr=uint16  SampleTime=-1
  Constant2 : Constant  Value=3  OutDataTypeStr=uint16  SampleTime=-1
  Constant3 : Constant  Value=3  OutDataTypeStr=uint16  SampleTime=-1
  HDL Counter : hdlsllib/Sources/HDL Counter  CountType=Free running  CountInit=0  CountStep=1  CountMax=25  CountFromType=Initial value  CountFrom=0  CountResetPort=on  CountLoadPort=off  CountEnbPort=on  CountDirPort=off  CountHitOutputPort=off  CountDataType=Unsigned  CountWordLen=16  CountFracLen=0  CountSampTime=1
  Logical Operator2 : Logic  IconShape=distinctive  AllPortsSameDT=off  OutDataTypeStr=boolean
  Logical Operator3 : Logic  Operator=NOT  IconShape=distinctive  AllPortsSameDT=off  OutDataTypeStr=boolean
  Logical Operator4 : Logic  Operator=NOT  IconShape=distinctive  AllPortsSameDT=off  OutDataTypeStr=boolean
  Logical Operator5 : Logic  IconShape=distinctive  AllPortsSameDT=off  OutDataTypeStr=boolean
  Relational Operator1 : RelationalOperator  Operator=<  OutDataTypeStr=boolean  InputSameDT=off
  Relational Operator2 : RelationalOperator  Operator=<  OutDataTypeStr=boolean  InputSameDT=off
  Relational Operator3 : RelationalOperator  Operator=<  OutDataTypeStr=boolean  InputSameDT=off
  falling_edge_detector : $bdroot/falling_edge_detector  SystemSampleTime=-1  VariantActivationTime=update diagram  AllowFlexibleInterface=on  Latency=0  AutoFrameSizeCalculation=off
  falling_edge_detector1 : $bdroot/falling_edge_detector  SystemSampleTime=-1  VariantActivationTime=update diagram  AllowFlexibleInterface=on  Latency=0  AutoFrameSizeCalculation=off
  rising_edge_detector1 : $bdroot/rising_edge_detector  SystemSampleTime=-1  VariantActivationTime=update diagram  AllowFlexibleInterface=on  Latency=0  AutoFrameSizeCalculation=off
  is_channel : Outport
  is_header : Outport  Port=2
  is_payload : Outport  Port=3
  last_frame : Outport  Port=4  VectorParamsAs1DForOutWhenUnconnected=off
  wires:
  Relational Operator3/1 -> Logical Operator5/2
  Constant3/1 -> Add/1
  Add/1 -> Relational Operator3/2
  payload_num_ofdm_symbols/1 -> Add/2
  falling_edge_detector/1 -> last_frame/1
  Logical Operator5/1 -> is_payload/1, falling_edge_detector/1  "payload"
  Logical Operator4/1 -> Logical Operator5/1  "payload"
  valid/1 -> falling_edge_detector1/1
  falling_edge_detector1/1 -> HDL Counter/2
  Constant1/1 -> Relational Operator1/2
  Constant2/1 -> Relational Operator2/2
  HDL Counter/1 -> Relational Operator1/1, Relational Operator2/1, Relational Operator3/1
  Relational Operator2/1 -> Logical Operator4/1, Logical Operator2/2
  Logical Operator3/1 -> Logical Operator2/1
  Logical Operator2/1 -> is_header/1  "header"
  Relational Operator1/1 -> Logical Operator3/1, is_channel/1  "channel"
  rst/1 -> rising_edge_detector1/1
  rising_edge_detector1/1 -> HDL Counter/1

== system HDL_ieee_8021513/rx_payload_full/next_frame_to_ready_rx ==
  note: Given a next frame rising edge, this subsystem will generate a "ready" signal for the duration of "payloadBitsPerFec" clock cycles
  next_frame : Inport
  HDL Counter : hdlsllib/Sources/HDL Counter  CountType=Count limited  CountInit=0  CountStep=1  CountMax=payloadBitsPerFec-1  CountFromType=Initial value  CountFrom=0  CountResetPort=off  CountLoadPort=off  CountEnbPort=on  CountDirPort=off  CountHitOutputPort=on  CountDataType=Unsigned  CountWordLen=nextpow2(payloadBitsPerFec)  CountFracLen=0  CountSampTime=1
  Logical Operator2 : Logic  Operator=NOT  IconShape=distinctive  AllPortsSameDT=off  OutDataTypeStr=boolean
  Logical Operator3 : Logic  Operator=OR  IconShape=distinctive  AllPortsSameDT=off  OutDataTypeStr=boolean
  Terminator : Terminator
  Unit Delay Enabled Synchronous : hdlsllib/Discrete/Unit Delay Enabled Synchronous  InitialCondition=0.0  SampleTime=-1
  rising_edge_detector : $bdroot/rising_edge_detector  SystemSampleTime=-1  VariantActivationTime=update diagram  AllowFlexibleInterface=on  Latency=0  AutoFrameSizeCalculation=off
  ready : Outport  VectorParamsAs1DForOutWhenUnconnected=off
  wires:
  rising_edge_detector/1 -> Logical Operator3/1
  Logical Operator2/1 -> Unit Delay Enabled Synchronous/1
  HDL Counter/1 -> Terminator/1
  Unit Delay Enabled Synchronous/1 -> HDL Counter/1, ready/1
  Logical Operator3/1 -> Unit Delay Enabled Synchronous/2
  HDL Counter/2 -> Logical Operator3/2, Logical Operator2/1
  next_frame/1 -> rising_edge_detector/1

== system HDL_ieee_8021513/rx_payload_full/reduced_ldpc_rx ==
  data_in : Inport
  ctrl_in : Inport  Port=2
  fec_rate : Inport  Port=3
  block_size : Inport  Port=4
  Hc_12S_B80 : whdledac/LDPC Decoder  ParityCheckMatrix=Hc_12S  BlockSize=80  Algorithm=Min-sum  ScalingFactor=0.75  Termination=Max  SpecifyInputs=Property  NumIterations=ldpcDecoderMaxNumberIterations  MaxNumIterations=8  ParityCheckStatus=off  SimulateUsing=Code generation
  Terminator : Terminator
  Terminator1 : Terminator
  data_out : Outport
  ctrl_out : Outport  Port=2
  next_frame : Outport  Port=3  VectorParamsAs1DForOutWhenUnconnected=off
  wires:
  Hc_12S_B80/1 -> data_out/1
  Hc_12S_B80/2 -> ctrl_out/1
  data_in/1 -> Hc_12S_B80/1
  ctrl_in/1 -> Hc_12S_B80/2
  fec_rate/1 -> Terminator/1
  block_size/1 -> Terminator1/1
  Hc_12S_B80/3 -> next_frame/1

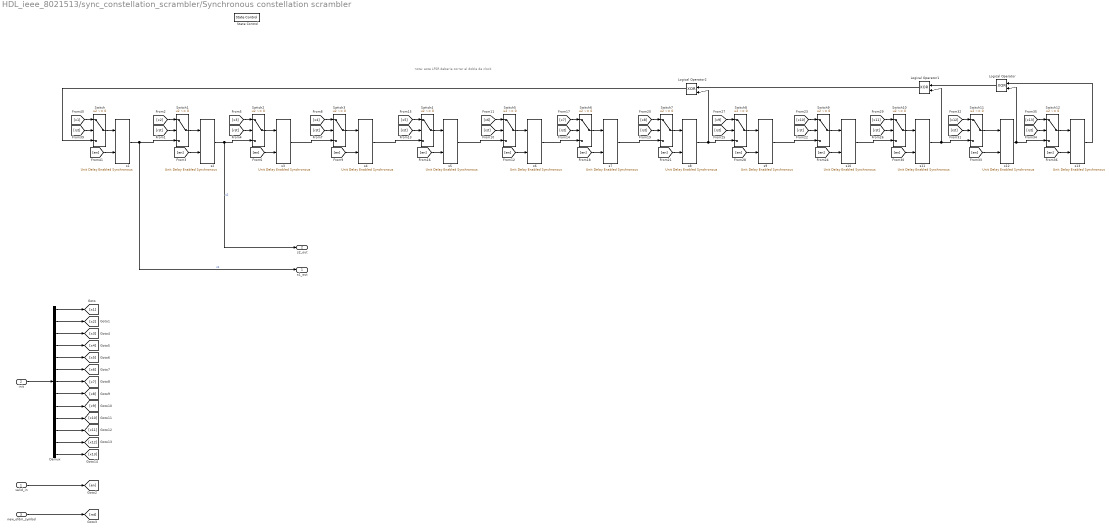
== system HDL_ieee_8021513/sync_constellation_scrambler/Synchronous constellation scrambler ==
  note: nota: este LFSR deberia correr al doble de clock
  valid_in : Inport
  init : Inport  Port=2
  new_ofdm_symbol : Inport  Port=3
  Demux : Demux  Outputs=13
  Logical Operator : Logic  Operator=XOR  IconShape=distinctive  AllPortsSameDT=off  OutDataTypeStr=boolean
  Logical Operator1 : Logic  Operator=XOR  IconShape=distinctive  AllPortsSameDT=off  OutDataTypeStr=boolean
  Logical Operator2 : Logic  Operator=XOR  IconShape=distinctive  AllPortsSameDT=off  OutDataTypeStr=boolean
  State Control : StateControl  StateControl=Synchronous
  Switch{,1..12} (13 alike) : Switch  Criteria=u2 ~= 0  SaturateOnIntegerOverflow=off  InputSameDT=off
  s{1..13} (13 alike) : hdlsllib/Discrete/Unit Delay Enabled Synchronous  InitialCondition=0.0  SampleTime=-1
  s1_out : Outport  VectorParamsAs1DForOutWhenUnconnected=off
  s2_out : Outport  Port=2  VectorParamsAs1DForOutWhenUnconnected=off
  wires:
  [en] -> s11/2
  Demux/5 -> [x5]
  Logical Operator1/1 -> Logical Operator2/1
  [rst] -> Switch2/2
  s3/1 -> Switch3/3
  [rst] -> Switch9/2
  [x5] -> Switch4/1
  s8/1 -> Switch8/3, Logical Operator2/2
  Demux/13 -> [x13]
  [en] -> s9/2
  s13/1 -> Logical Operator/1
  Switch6/1 -> s7/1
  [en] -> s8/2
  [x9] -> Switch8/1
  [x2] -> Switch1/1
  s4/1 -> Switch4/3
  [rst] -> Switch/2
  Switch8/1 -> s9/1
  [x4] -> Switch3/1
  Switch12/1 -> s13/1
  [en] -> s7/2
  init/1 -> Demux/1
  [en] -> s4/2
  Switch7/1 -> s8/1
  s2/1 -> s2_out/1, Switch2/3  "s2"
  [rst] -> Switch11/2
  s9/1 -> Switch9/3
  [en] -> s5/2
  Demux/10 -> [x10]
  [en] -> s12/2
  Switch9/1 -> s10/1
  Switch1/1 -> s2/1
  s12/1 -> Switch12/3, Logical Operator/2
  [x7] -> Switch6/1
  Switch11/1 -> s12/1
  [rst] -> Switch6/2
  [en] -> s3/2
  [en] -> s2/2
  Demux/4 -> [x4]
  [x3] -> Switch2/1
  [en] -> s1/2
  Demux/2 -> [x2]
  valid_in/1 -> [en]
  [en] -> s6/2
  s6/1 -> Switch6/3
  Switch5/1 -> s6/1
  [rst] -> Switch12/2
  [x10] -> Switch9/1
  Logical Operator2/1 -> Switch/3
  [rst] -> Switch7/2
  Demux/11 -> [x11]
  Switch/1 -> s1/1
  Switch4/1 -> s5/1
  [rst] -> Switch5/2
  [x6] -> Switch5/1
  [x11] -> Switch10/1
  Logical Operator/1 -> Logical Operator1/1
  s5/1 -> Switch5/3
  s11/1 -> Switch11/3, Logical Operator1/2
  [x1] -> Switch/1
  Demux/9 -> [x9]
  s10/1 -> Switch10/3
  new_ofdm_symbol/1 -> [rst]
  [rst] -> Switch3/2
  [en] -> s13/2
  [rst] -> Switch1/2
  [x12] -> Switch11/1
  [rst] -> Switch8/2
  [en] -> s10/2
  Switch2/1 -> s3/1
  Demux/3 -> [x3]
  Demux/7 -> [x7]
  [rst] -> Switch4/2
  Demux/8 -> [x8]
  Demux/1 -> [x1]
  Demux/12 -> [x12]
  Demux/6 -> [x6]
  Switch3/1 -> s4/1
  s1/1 -> s1_out/1, Switch1/3  "s1"
  [rst] -> Switch10/2
  [x8] -> Switch7/1
  s7/1 -> Switch7/3
  Switch10/1 -> s11/1
  [x13] -> Switch12/1

== system HDL_ieee_8021513/constellation_descrambler/rotate_-90/rotate_-90 ==
  s2 : Inport
  s1 : Inport  Port=2
  data_in : Inport  Port=3
  Bit Concat : hdlsllib/Logic and Bit Operations/Bit Concat  numInputs=2
  Complex to Real-Imag : ComplexToRealImag
  Complex to Real-Imag1 : ComplexToRealImag
  Complex to Real-Imag2 : ComplexToRealImag
  Multiport Switch : MultiPortSwitch  DataPortOrder=Zero-based contiguous  Inputs=4  zeroidx=on  SaturateOnIntegerOverflow=off  InputSameDT=off
  Real-Imag to Complex : RealImagToComplex
  Real-Imag to Complex1 : RealImagToComplex
  Real-Imag to Complex2 : RealImagToComplex
  Unary Minus{,1..3} (4 alike) : UnaryMinus
  data_out : Outport
  wires:
  Unary Minus3/1 -> Real-Imag to Complex/2
  Multiport Switch/1 -> data_out/1
  Real-Imag to Complex2/1 -> Multiport Switch/5
  Complex to Real-Imag2/1 -> Real-Imag to Complex2/2
  Real-Imag to Complex1/1 -> Multiport Switch/3
  Complex to Real-Imag1/2 -> Real-Imag to Complex1/1
  Real-Imag to Complex/1 -> Multiport Switch/4
  Complex to Real-Imag/2 -> Unary Minus3/1
  Unary Minus/1 -> Real-Imag to Complex/1
  Complex to Real-Imag/1 -> Unary Minus/1
  data_in/1 -> Multiport Switch/2, Complex to Real-Imag/1, Complex to Real-Imag2/1, Complex to Real-Imag1/1
  Bit Concat/1 -> Multiport Switch/1
  s1/1 -> Bit Concat/2
  s2/1 -> Bit Concat/1
  Complex to Real-Imag1/1 -> Unary Minus1/1
  Unary Minus1/1 -> Real-Imag to Complex1/2
  Complex to Real-Imag2/2 -> Unary Minus2/1
  Unary Minus2/1 -> Real-Imag to Complex2/1

== system HDL_ieee_8021513/full_rx/prepare_payload_data/payload_clock_x2 ==
  data_in : Inport
  valid_in : Inport  Port=2
  Demux : Demux
  Serializer1D : hdlsllib/HDL Operations/Serializer1D  Ratio=2  IdleCycles=0  validIn=on  startOut=off  validOut=on  inputDataDimensions=-1  inputSampleTime=-1  inputSignalType=auto
  Terminator : Terminator
  Terminator1 : Terminator
  Vector Concatenate : Concatenate  Mode=Multidimensional array
  data_out : Outport
  valid_out : Outport  Port=2
  wires:
  Demux/3 -> Vector Concatenate/1
  Demux/1 -> Terminator/1
  data_in/1 -> Demux/1
  Demux/2 -> Terminator1/1
  Serializer1D/1 -> data_out/1
  Serializer1D/2 -> valid_out/1
  valid_in/1 -> Serializer1D/2
  Demux/4 -> Vector Concatenate/2
  Vector Concatenate/1 -> Serializer1D/1  "paralel_dataIn"

== system HDL_ieee_8021513/full_tx/store_frame_in_ram/RAM ==
  new_din : Inport
  new_wr_addr : Inport  Port=2
  new_we : Inport  Port=3
  new_rd_addr : Inport  Port=4
  Simple Dual Port RAM System : hdlsllib/HDL RAMs/Simple Dual Port RAM System  RAMType=Simple dual port  AsyncRead=off  WriteOutputValue=New data  RAMInitialValue=0  allowBusInputs=off  WritesHaveOutput=on  NumReads=0  NumWrites=1  SimulateUsing=Code generation
  dout_new : Outport
  wires:
  new_wr_addr/1 -> Simple Dual Port RAM System/2
  new_we/1 -> Simple Dual Port RAM System/3
  new_din/1 -> Simple Dual Port RAM System/1
  Simple Dual Port RAM System/1 -> dout_new/1  "dout_new"
  new_rd_addr/1 -> Simple Dual Port RAM System/4
